simulink model "Refined_Model_3"  (R2020b)
settings: Solver=FixedStepAuto  StartTime=0.0  StopTime=90  FixedStep=dt  RelTol=1e-3
values from neighbouring files (symbols this model uses):
  CovDist = RoadProfile(:,4)    [ICE_Val.m]
  Cx = VehicleDefine(7,3)    [BEV_Basictest.m]    (also in GPS_val.m; ICEBEV_Script.m; ICEBEV_Script_VECTO.m; ICE_Script.m)
  DynRolRad = VehicleDefine(5,3)    [BEV_Basictest.m]    (also in GPS_val.m; ICEBEV_Script.m; ICEBEV_Script_VECTO.m; ICE_Script.m)
  EngineRpm = round(IntpTorCur(:,1))    [GPS_val.m]    (also in ICEBEV_Script.m; ICEBEV_Script_VECTO.m; ICE_Script.m; ICE_Script_SSVal.m)
  etaClutch = VehicleDefine(23,3)    [GPS_val.m]    (also in ICEBEV_Script.m; ICEBEV_Script_VECTO.m; ICE_Script.m; ICE_Script_SSVal.m)
  etaGRa = GBXDefine(:,3)    [GPS_val.m]    (also in ICEBEV_Script.m; ICEBEV_Script_VECTO.m; ICE_Script.m; ICE_Script_SSVal.m)
  FCTableVal = FCMap(2:end,2:end)    [GPS_val.m]    (also in ICEBEV_Script.m; ICEBEV_Script_VECTO.m; ICE_Script.m; ICE_Script_SSVal.m)
  FDR = VehicleDefine(20,3)    [BEV_Basictest.m]    (also in GPS_val.m = VehicleDefine(22,3); ICEBEV_Script.m = VehicleDefine(22,3); ICEBEV_Script_VECTO.m = VehicleDefine(22,3); ICE_Script.m = VehicleDefine(22,3))
  FLoadTor = IntpTorCur(:,2)    [GPS_val.m]    (also in ICEBEV_Script.m; ICEBEV_Script_VECTO.m; ICE_Script.m; ICE_Script_SSVal.m)
  Fr = VehicleDefine(13,3)    [BEV_Basictest.m]    (also in GPS_val.m; ICEBEV_Script.m; ICEBEV_Script_VECTO.m; ICE_Script.m)
  g = VehicleDefine(14,3)    [BEV_Basictest.m]    (also in GPS_val.m; ICEBEV_Script.m; ICEBEV_Script_VECTO.m; ICE_Script.m)
  GNo = GBXDefine(:,1)    [GPS_val.m]    (also in ICEBEV_Script.m; ICEBEV_Script_VECTO.m; ICE_Script.m; ICE_Script_SSVal.m)
  GRa = GBXDefine(:,2)    [GPS_val.m]    (also in ICEBEV_Script.m; ICEBEV_Script_VECTO.m; ICE_Script.m; ICE_Script_SSVal.m)
  InitVel = VehicleDefine(21,3)    [BEV_Basictest.m]    (also in GPS_val.m = VehicleDefine(24,3); ICEBEV_Script.m = VehicleDefine(24,3); ICEBEV_Script_VECTO.m = VehicleDefine(24,3); ICE_Script.m = VehicleDefine(24,3))
  IntpSlope = round(IntpSlope,1)    [GPS_val.m]    (also in ICE_Script.m; ICE_Val.m = A)
  Je = VehicleDefine(25,3)    [GPS_val.m]    (also in ICEBEV_Script.m; ICEBEV_Script_VECTO.m; ICE_Script.m; ICE_Script_SSVal.m)
  Jk = VehicleDefine(15,3)    [BEV_Basictest.m]    (also in GPS_val.m; ICEBEV_Script.m; ICEBEV_Script_VECTO.m; ICE_Script.m)
  Jm = VehicleDefine(16,3)    [GPS_val.m]    (also in ICEBEV_Script.m; ICEBEV_Script_VECTO.m; ICE_Script.m; ICE_Script_SSVal.m)
  MaxDec = 1    [BEV_Basictest.m]    (also in GPS_val.m; ICEBEV_Script.m; ICEBEV_Script_VECTO.m; ICE_Script.m)
  MaxSpeedProfile = FMSP    [GPS_val.m]    (also in ICE_Script.m; ICE_Val.m = repelem(SegSPLatinmps,SegLeninm))
  Me = VehicleDefine(10,3)    [BEV_Basictest.m]    (also in GPS_val.m; ICEBEV_Script.m; ICEBEV_Script_VECTO.m; ICE_Script.m)
  MotoringTor = IntpTorCur(:,3)    [GPS_val.m]    (also in ICEBEV_Script.m; ICEBEV_Script_VECTO.m; ICE_Script.m; ICE_Script_SSVal.m)
  Mt = VehicleDefine(12,3)    [BEV_Basictest.m]    (also in GPS_val.m; ICEBEV_Script.m; ICEBEV_Script_VECTO.m; ICE_Script.m)
  Mtot = Mv+Me+Mt    [BEV_Basictest.m]    (also in GPS_val.m; ICEBEV_Script.m; ICEBEV_Script_VECTO.m; ICE_Script.m)
  Mv = VehicleDefine(9,3)    [BEV_Basictest.m]    (also in GPS_val.m; ICEBEV_Script.m; ICEBEV_Script_VECTO.m; ICE_Script.m)
  NoSteps = round(Dist(end))    [GPS_val.m]    (also in ICE_Script.m; ICE_Val.m = 3002)
  NoWhlFA = VehicleDefine(2,3)    [BEV_Basictest.m]    (also in GPS_val.m; ICE_Script.m; ICE_Val.m; ICE_Val_new.m)
  NoWhlRA = VehicleDefine(4,3)    [BEV_Basictest.m]    (also in GPS_val.m; ICE_Script.m; ICE_Val.m; ICE_Val_new.m)
  rho = VehicleDefine(6,3)    [BEV_Basictest.m]    (also in GPS_val.m; ICEBEV_Script.m; ICEBEV_Script_VECTO.m; ICE_Script.m)
  RpmBrkPnt = ThrottleMap(1,:)    [GPS_val.m]    (also in ICEBEV_Script.m; ICEBEV_Script_VECTO.m; ICE_Script.m; ICE_Script_SSVal.m)
  s = divisors(length(MaxSpeedProfile))    [GPS_val.m]    (also in ICEBEV_Script.m = round(FLoadTor); ICEBEV_Script_VECTO.m = round(FLoadTor); ICE_Script.m = round(FLoadTor); ICE_Script_SSVal.m = round(FLoadTor))
  SegNo = RoadProfile(:,1)    [ICE_Val.m]
  SegSPLatinmps = (sqrt(aMaxLat*g*CurRadinm))    [GPS_val.m]    (also in ICE_Script.m; ICE_Val.m)
  Sx = VehicleDefine(8,3)    [BEV_Basictest.m]    (also in GPS_val.m; ICEBEV_Script.m; ICEBEV_Script_VECTO.m; ICE_Script.m)
  ThrotPos = ThrotPos'    [GPS_val.m]    (also in ICEBEV_Script.m; ICEBEV_Script_VECTO.m; ICE_Script.m; ICE_Script_SSVal.m)
  ThrotTableVal = ThrottleMap(2:end,2:end)    [GPS_val.m]    (also in ICEBEV_Script.m; ICEBEV_Script_VECTO.m; ICE_Script.m; ICE_Script_SSVal.m)
undefined symbols (not defined in the file or in its folder): Ftractive, G1Inprpm, GearNo, GInprpm, GInpTor, GTorLoss, MaxSpinG, MaxWhlTorinG
libraries: simulink x4, simulink_extras x2, autolibshared x1
settings Model: Creator=Kshitij  LastModifiedBy=Kshitij
settings DebuggingCC: AlgebraicLoopMsg=none

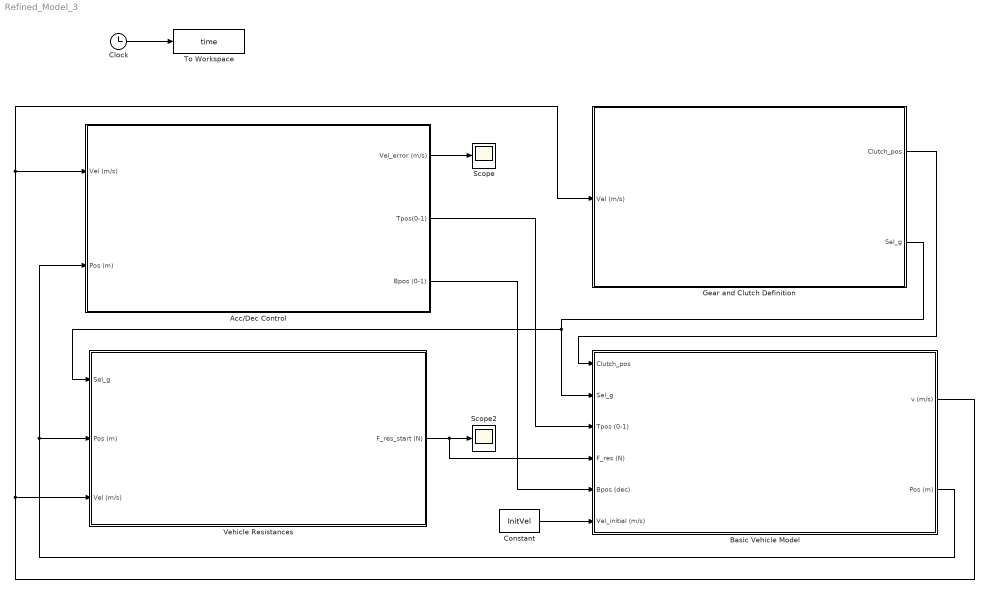
== system Refined_Model_3 ==
  Acc/Dec Control : Subsystem
  Basic Vehicle Model : Subsystem
  Clock : Clock
  Constant : Constant  Value=InitVel
  Gear and Clutch Definition : Subsystem
  Scope : Scope
  Scope2 : Scope
  To Workspace : ToWorkspace  VariableName=time  SaveFormat=Timeseries  SampleTime=-1
  Vehicle Resistances : Subsystem
  wires:
  Vehicle Resistances/1(F_res_start (N)) -> Basic Vehicle Model/4(F_res (N)), Scope2/1
  Basic Vehicle Model/2(Pos (m)) -> Acc/Dec Control/2(Pos (m)), Vehicle Resistances/2(Pos (m))
  Basic Vehicle Model/1(v (m/s)) -> Vehicle Resistances/3(Vel (m/s)), Gear and Clutch Definition/1(Vel (m/s)), Acc/Dec Control/1(Vel (m/s))
  Constant/1 -> Basic Vehicle Model/6(Vel_initial (m/s))
  Acc/Dec Control/1(Vel_error (m/s)) -> Scope/1
  Gear and Clutch Definition/2(Sel_g) -> Basic Vehicle Model/2(Sel_g), Vehicle Resistances/1(Sel_g)
  Gear and Clutch Definition/1(Clutch_pos) -> Basic Vehicle Model/1(Clutch_pos)
  Clock/1 -> To Workspace/1
  Acc/Dec Control/2(Tpos(0-1)) -> Basic Vehicle Model/3(Tpos (0-1))
  Acc/Dec Control/3(Bpos (0-1)) -> Basic Vehicle Model/5(Bpos (dec))

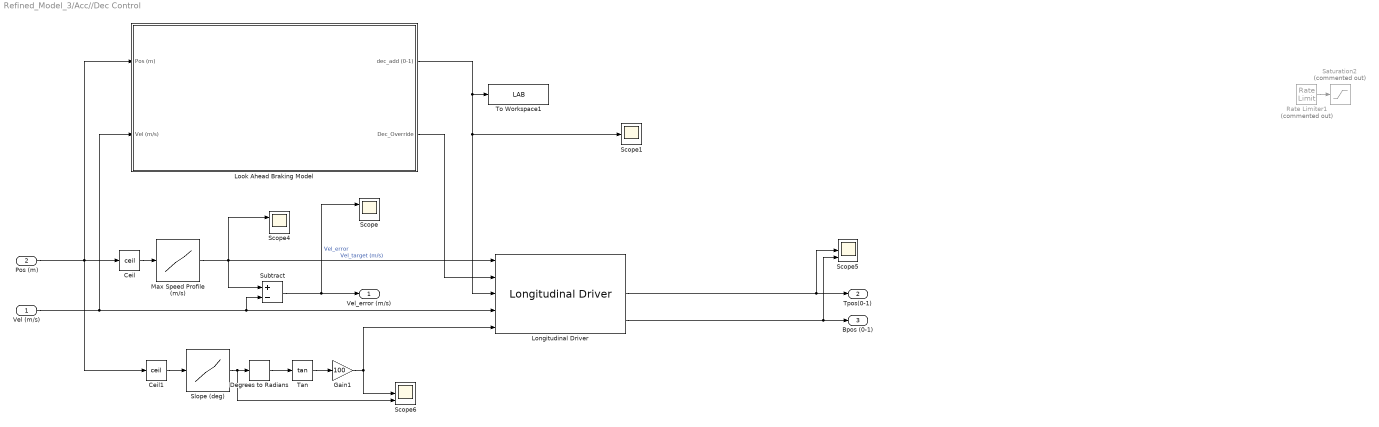
== system Refined_Model_3/Acc//Dec Control ==
  Vel (m/s) : Inport
  Pos (m) : Inport  Port=2
  Ceil : Rounding  Operator=ceil
  Ceil1 : Rounding  Operator=ceil
  Degrees to Radians : simulink_extras/Transformations/Degrees to Radians
  Gain1 : Gain  Gain=100
  Longitudinal Driver : autolibshared/Longitudinal Driver  extAccelOvr=off  extDecelOvr=on  extAccelHld=off  extDecelHld=off  extAccelZero=off  extDecelZero=off  cntrlType=PI  shftType=None  velUnits=m/s  gearOut=off  Kp=10  Ki=20  Kff=.05  Kg=.01  VehVelVec=[0 100]  KffVec=[.1 .1]  KpVec=[10 10]  KiVec=[5 5]  KgVec=[0 0]  m=1500  Kpt=3000  tau=.1  L=2  aR=200  bR=2.5  cR=.5  g=9.81  vnom=100  Kaw=.1  tauerr=.03  tauPt=2  GearInit=0  tShift=.1  pdlVec=[0.1 0.4 0.5 0.9]  upShftTbl=[-1 12.9375 26.4375 39.9375 51.18749999999999 62.4375 72.84375 83.25;-1 16.3125 29.8125 43.3125 54.5624 65.8125 76.78125 87.75;-1 19.6875 33.1875 46.68749999999999 57.9375 69.1875 80.71875 92.25;-1 33 52.5 77.25 100.5 138.75 161.875 185]  dwnShftTbl=[1 9.5625 23.0625 36.5625 47.8125 59.0625 68.90625 78.75;1 12.9375 26.4375 39.9375 51.18749999999999 62.4375 72.84375 83.25;1 16.3125 29.8125 43.3125 54.562499 65.8125 76.78125 87.75;1 19.6875 33.1875 46.68749999999999 57.9375 69.1875 80.71875 92.25]  tClutch=.5  tRev=.5  tPark=120  aMode=1  UpGearVec="[0  1  2  3  4  5  6  7]"  DownGearVec="[1  2  3  4  5  6  7  8]"
      settings: SourceProductBaseCode=PW,MT,UV,VE,VP
  Look Ahead Braking Model : Subsystem
  Max Speed Profile (m/s) : Lookup_n-D  NumberOfTableDimensions=1  BreakpointsForDimension1=[1:length(MaxSpeedProfile)]  BreakpointsForDimension2=G1Inprpm  Table=MaxSpeedProfile  InterpMethod=Linear Lagrange  InternalRulePriority=Speed  RndMeth=Simplest  InputSameDT=on
  Rate Limiter1 : RateLimiter  Commented=on  RisingSlewLimit=0.5  FallingSlewLimit=-0.5  SampleTimeMode=inherited
  Saturation2 : Saturate  Commented=on  UpperLimit=1  LowerLimit=-1
  Scope : Scope  NumInputPorts=2
  Scope1 : Scope
  Scope4 : Scope  NumInputPorts=2
  Scope5 : Scope  NumInputPorts=3
  Scope6 : Scope  NumInputPorts=3
  Slope (deg) : Lookup_n-D  NumberOfTableDimensions=1  BreakpointsForDimension1=1: length(IntpSlope)  Table=IntpSlope  InternalRulePriority=Speed  RndMeth=Simplest  InputSameDT=on
  Subtract : Sum  Inputs=+-
  Tan : Trigonometry  Operator=tan
  To Workspace1 : ToWorkspace  VariableName=LAB  SaveFormat=Timeseries  SampleTime=-1
  Vel_error (m/s) : Outport
  Tpos(0-1) : Outport  Port=2
  Bpos (0-1) : Outport  Port=3
  wires:
  Max Speed Profile (m/s)/1 -> Subtract/1, Longitudinal Driver/1, Scope4/1  "Vel_target (m/s)"
  Subtract/1 -> Scope/1, Vel_error (m/s)/1  "Vel_error"
  Ceil/1 -> Max Speed Profile (m/s)/1
  Look Ahead Braking Model/1(dec_add (0-1)) -> Longitudinal Driver/3, Scope1/1, To Workspace1/1
  Pos (m)/1 -> Ceil1/1, Ceil/1, Look Ahead Braking Model/1(Pos (m))
  Rate Limiter1/1 -> Saturation2/1
  Vel (m/s)/1 -> Longitudinal Driver/4, Subtract/2, Look Ahead Braking Model/2(Vel (m/s))
  Slope (deg)/1 -> Scope6/3, Degrees to Radians/1
  Ceil1/1 -> Slope (deg)/1
  Degrees to Radians/1 -> Tan/1
  Tan/1 -> Gain1/1
  Gain1/1 -> Scope6/2, Longitudinal Driver/5
  Longitudinal Driver/2 -> Scope5/2, Tpos(0-1)/1
  Longitudinal Driver/3 -> Scope5/3, Bpos (0-1)/1
  Look Ahead Braking Model/2(Dec_Override) -> Longitudinal Driver/2

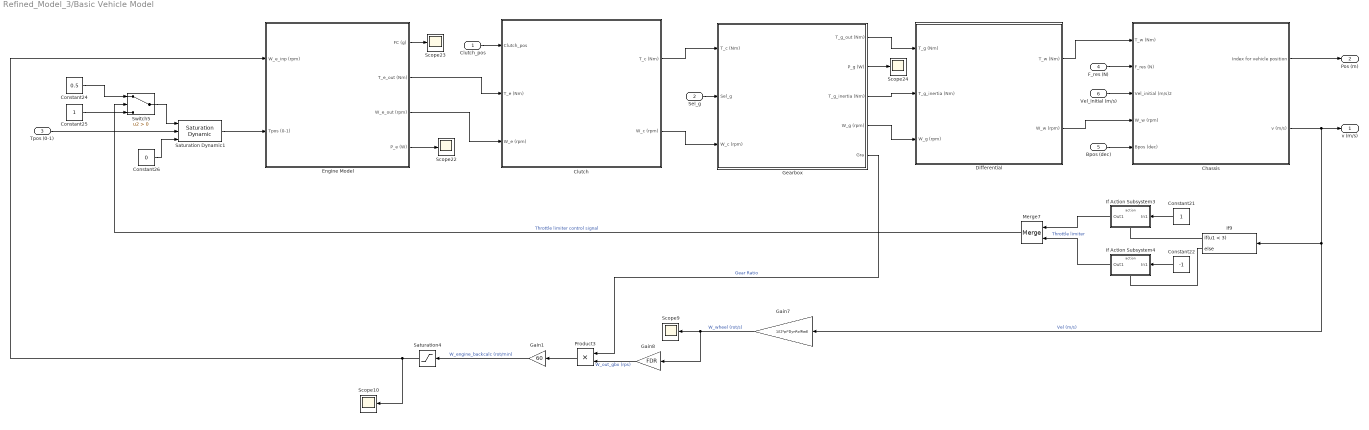
== system Refined_Model_3/Basic Vehicle Model ==
  Clutch_pos : Inport
  Sel_g : Inport  Port=2
  Tpos (0-1) : Inport  Port=3
  F_res (N) : Inport  Port=4
  Bpos (dec) : Inport  Port=5
  Vel_initial (m/s) : Inport  Port=6
  Chassis : Subsystem
  Clutch : Subsystem
  Constant21 : Constant
  Constant22 : Constant  Value=-1
  Constant24 : Constant  Value=0.5
  Constant25 : Constant
  Constant26 : Constant  Value=0
  Differential : Subsystem
  Engine Model : Subsystem
  Gain1 : Gain  Gain=60
  Gain7 : Gain  Gain=1/(2*pi*DynRolRad)
  Gain8 : Gain  Gain=FDR
  Gearbox : Subsystem
  If Action Subsystem3 : Subsystem  TreatAsAtomicUnit=on
  If Action Subsystem4 : Subsystem  TreatAsAtomicUnit=on
  If9 : If  IfExpression=u1 < 3
  Merge7 : Merge
  Product3 : Product
  Saturation Dynamic1 : simulink/Discontinuities/Saturation Dynamic  OutMin=[]  OutMax=[]  OutDataTypeStr=Inherit: Same as second input  OutDataType=fixdt(1, 16)  OutScaling=2^-10  DoSatur=off
  Saturation4 : Saturate  UpperLimit=max(EngineRpm)  LowerLimit=min(EngineRpm)
  Scope{9..10,22..24} (5 alike) : Scope
  Switch5 : Switch  Criteria=u2 > Threshold
  v (m/s) : Outport
  Pos (m) : Outport  Port=2
  wires:
  Gearbox/1(T_g_out (Nm)) -> Differential/1(T_g (Nm))
  Gearbox/4(W_g (rpm)) -> Differential/3(W_g (rpm))
  Gearbox/3(T_g_inertia (Nm)) -> Differential/2(T_g_inertia (Nm))
  Chassis/1(Index for vehicle position) -> Pos (m)/1
  Bpos (dec)/1 -> Chassis/5(Bpos (dec))
  Vel_initial (m/s)/1 -> Chassis/3(Vel_initial (m/s)2)
  Differential/1(T_w (Nm)) -> Chassis/1(T_w (Nm))
  F_res (N)/1 -> Chassis/2(F_res (N))
  Constant21/1 -> If Action Subsystem3/1(In1)
  If9/1 -> If Action Subsystem3/Action
  Gearbox/2(P_g (W)) -> Scope24/1
  Clutch/1(T_c (Nm)) -> Gearbox/1(T_c (Nm))
  Clutch/2(W_c (rpm)) -> Gearbox/3(W_c (rpm))
  Saturation Dynamic1/1 -> Engine Model/2(Tpos (0-1))
  Tpos (0-1)/1 -> Saturation Dynamic1/2
  Merge7/1 -> Switch5/2  "Throttle limiter control signal"
  Constant26/1 -> Saturation Dynamic1/3
  Constant24/1 -> Switch5/1
  Engine Model/4(P_e (W)) -> Scope22/1
  Constant25/1 -> Switch5/3
  If Action Subsystem3/1(Out1) -> Merge7/1
  Switch5/1 -> Saturation Dynamic1/1
  Differential/2(W_w (rpm)) -> Chassis/4(W_w (rpm))
  Engine Model/2(T_e_out (Nm)) -> Clutch/2(T_e (Nm))
  Engine Model/1(FC (g)) -> Scope23/1
  Sel_g/1 -> Gearbox/2(Sel_g)
  If9/2 -> If Action Subsystem4/Action
  Engine Model/3(W_e_out (rpm)) -> Clutch/3(W_e (rpm))
  If Action Subsystem4/1(Out1) -> Merge7/2  "Throttle limiter"
  Clutch_pos/1 -> Clutch/1(Clutch_pos)
  Constant22/1 -> If Action Subsystem4/1(In1)
  Gain1/1 -> Saturation4/1  "W_engine_backcalc (rot/min)"
  Gain7/1 -> Scope9/1, Gain8/1  "W_wheel (rot/s)"
  Chassis/2(v (m/s)) -> v (m/s)/1, Gain7/1, If9/1  "Vel (m/s)"
  Gearbox/5(Gra) -> Product3/1  "Gear Ratio"
  Product3/1 -> Gain1/1
  Gain8/1 -> Product3/2  "W_out_gbx (rps)"
  Saturation4/1 -> Scope10/1, Engine Model/1(W_e_inp (rpm))

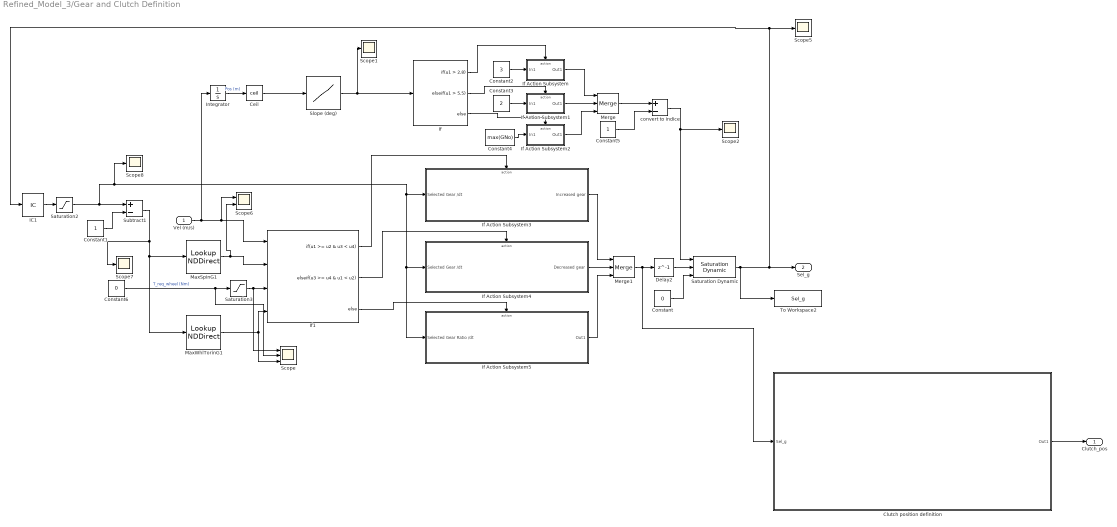
== system Refined_Model_3/Gear and Clutch Definition ==
  Vel (m/s) : Inport
  Ceil : Rounding  Operator=ceil
  Clutch position definition : Subsystem
  Constant : Constant  Value=0
  Constant1 : Constant
  Constant2 : Constant  Value=3
  Constant3 : Constant  Value=2
  Constant4 : Constant  Value=max(GNo)
  Constant5 : Constant
  Constant6 : Constant  Value=0
  Delay2 : Delay  DelayLength=1
  IC1 : InitialCondition
  If : If  IfExpression=u1 > 2.8  ElseIfExpressions=u1 > 5.5
  If Action Subsystem : Subsystem  TreatAsAtomicUnit=on
  If Action Subsystem1 : Subsystem  TreatAsAtomicUnit=on
  If Action Subsystem2 : Subsystem  TreatAsAtomicUnit=on
  If Action Subsystem3 : Subsystem  TreatAsAtomicUnit=on
  If Action Subsystem4 : Subsystem  TreatAsAtomicUnit=on
  If Action Subsystem5 : Subsystem  TreatAsAtomicUnit=on
  If1 : If  NumInputs=4  IfExpression=u1 >= u2 & u3 < u4  ElseIfExpressions=u3 >= u4 & u1 < u2
  Integrator : Integrator
  MaxSpinG1 : LookupNDDirect  NumberOfTableDimensions=1  Table=MaxSpinG
  MaxWhlTorinG1 : LookupNDDirect  NumberOfTableDimensions=1  Table=MaxWhlTorinG
  Merge : Merge  Inputs=3
  Merge1 : Merge  Inputs=3
  Saturation Dynamic : simulink/Discontinuities/Saturation Dynamic  OutMin=[]  OutMax=[]  OutDataTypeStr=Inherit: Same as second input  OutDataType=fixdt(1, 16)  OutScaling=2^-10  DoSatur=off
  Saturation2 : Saturate  UpperLimit=max(GNo)  LowerLimit=0
  Saturation3 : Saturate  UpperLimit=inf  LowerLimit=0
  Scope : Scope  NumInputPorts=3
  Scope{1..2,5,7..8} (5 alike) : Scope
  Scope6 : Scope  NumInputPorts=2
  Slope (deg) : Lookup_n-D  NumberOfTableDimensions=1  BreakpointsForDimension1=1: length(IntpSlope)  Table=IntpSlope  InternalRulePriority=Speed  RndMeth=Simplest  InputSameDT=on
  Subtract1 : Sum  Inputs=+-
  To Workspace2 : ToWorkspace  VariableName=Sel_g  SaveFormat=Timeseries  SampleTime=-1
  convert to indice : Sum  Inputs=+-
  Clutch_pos : Outport
  Sel_g : Outport  Port=2
  wires:
  IC1/1 -> Saturation2/1
  Merge1/1 -> Clutch position definition/1(Sel_g), Delay2/1
  Clutch position definition/1(Out1) -> Clutch_pos/1
  If1/2 -> If Action Subsystem4/Action
  If Action Subsystem4/1(Decreased gear) -> Merge1/2
  If1/3 -> If Action Subsystem5/Action
  If Action Subsystem3/1(Increased gear) -> Merge1/1
  Constant1/1 -> Subtract1/2
  MaxSpinG1/1 -> Scope6/2, If1/2
  If Action Subsystem5/1(Out1) -> Merge1/3
  Subtract1/1 -> Scope7/1, MaxSpinG1/1, MaxWhlTorinG1/1
  MaxWhlTorinG1/1 -> Scope/3, If1/4
  Saturation2/1 -> Subtract1/1, If Action Subsystem5/1(Selected Gear Ratio /dt), If Action Subsystem4/1(Selected Gear /dt), If Action Subsystem3/1(Selected Gear /dt), Scope8/1
  Vel (m/s)/1 -> If1/1, Scope6/1, Integrator/1
  If1/1 -> If Action Subsystem3/Action
  Saturation3/1 -> If1/3, Scope/1
  Integrator/1 -> Ceil/1  "Pos (m)"
  Ceil/1 -> Slope (deg)/1
  Slope (deg)/1 -> Scope1/1, If/1
  If/1 -> If Action Subsystem/Action
  If/2 -> If Action Subsystem1/Action
  Constant/1 -> Saturation Dynamic/3
  Constant2/1 -> If Action Subsystem/1(In1)
  If Action Subsystem/1(Out1) -> Merge/1
  If Action Subsystem1/1(Out1) -> Merge/2
  If/3 -> If Action Subsystem2/Action
  Constant3/1 -> If Action Subsystem1/1(In1)
  Constant4/1 -> If Action Subsystem2/1(In1)
  If Action Subsystem2/1(Out1) -> Merge/3
  convert to indice/1 -> Scope2/1, Saturation Dynamic/1
  Saturation Dynamic/1 -> To Workspace2/1, Sel_g/1, IC1/1, Scope5/1
  Delay2/1 -> Saturation Dynamic/2
  Merge/1 -> convert to indice/1
  Constant5/1 -> convert to indice/2
  Constant6/1 -> Scope/2, Saturation3/1  "T_req_wheel (Nm)"

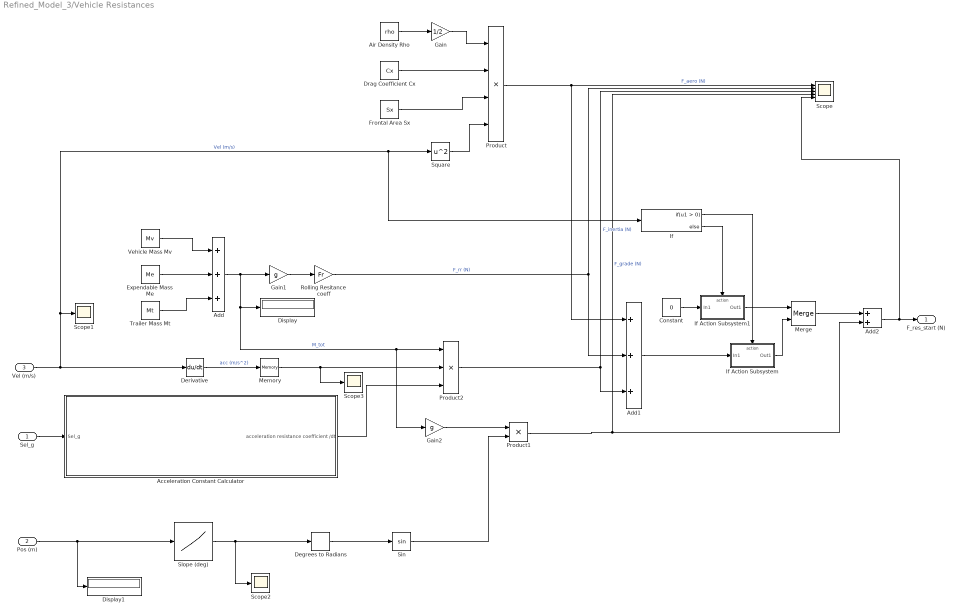
== system Refined_Model_3/Vehicle Resistances ==
  Sel_g : Inport
  Pos (m) : Inport  Port=2
  Vel (m/s) : Inport  Port=3
  Acceleration Constant Calculator : Subsystem
  Add : Sum  Inputs=+++
  Add1 : Sum  Inputs=+++
  Add2 : Sum
  Air Density Rho : Constant  Value=rho
  Constant : Constant  Value=0
  Degrees to Radians : simulink_extras/Transformations/Degrees to Radians
  Derivative : Derivative
  Display : Display
  Display1 : Display
  Drag Coefficient Cx : Constant  Value=Cx
  Expendable Mass Me : Constant  Value=Me
  Frontal Area Sx : Constant  Value=Sx
  Gain : Gain  Gain=1/2
  Gain1 : Gain  Gain=g
  Gain2 : Gain  Gain=g
  If : If
  If Action Subsystem : Subsystem  TreatAsAtomicUnit=on
  If Action Subsystem1 : Subsystem  TreatAsAtomicUnit=on
  Memory : Memory
  Merge : Merge
  Product : Product  Inputs=4
  Product1 : Product
  Product2 : Product  Inputs=3
  Rolling Resitance coeff : Gain  Gain=Fr
  Scope : Scope  NumInputPorts=5
  Scope1 : Scope
  Scope2 : Scope
  Scope3 : Scope
  Sin : Trigonometry
  Slope (deg) : Lookup_n-D  NumberOfTableDimensions=1  BreakpointsForDimension1=1: length(IntpSlope)  Table=IntpSlope  InternalRulePriority=Speed  RndMeth=Simplest  InputSameDT=on
  Square : Math  Operator=square  SaturateOnIntegerOverflow=on
  Trailer Mass Mt : Constant  Value=Mt
  Vehicle Mass Mv : Constant  Value=Mv
  F_res_start (N) : Outport
  wires:
  Expendable Mass Me/1 -> Add/2
  Add/1 -> Display/1, Product2/1, Gain2/1, Gain1/1  "M_tot"
  Gain/1 -> Product/1
  Sin/1 -> Product1/2
  Slope (deg)/1 -> Degrees to Radians/1, Scope2/1
  Product1/1 -> Add2/2, Scope/4  "F_grade (N)"
  Air Density Rho/1 -> Gain/1
  Drag Coefficient Cx/1 -> Product/2
  Vel (m/s)/1 -> Derivative/1, If/1, Square/1, Scope1/1  "Vel (m/s)"
  Pos (m)/1 -> Display1/1, Slope (deg)/1
  Gain2/1 -> Product1/1
  Trailer Mass Mt/1 -> Add/3
  Rolling Resitance coeff/1 -> Scope/2, Add1/2  "F_rr (N)"
  Square/1 -> Product/4
  Gain1/1 -> Rolling Resitance coeff/1
  Vehicle Mass Mv/1 -> Add/1
  Product/1 -> Add1/1, Scope/1  "F_aero (N)"
  Frontal Area Sx/1 -> Product/3
  Product2/1 -> Add1/3, Scope/3  "F_inertia (N)"
  Acceleration Constant Calculator/1(acceleration resistance coefficient /dt) -> Product2/3
  Sel_g/1 -> Acceleration Constant Calculator/1(Sel_g)
  Derivative/1 -> Memory/1  "acc (m/s^2)"
  If/1 -> If Action Subsystem/Action
  If/2 -> If Action Subsystem1/Action
  If Action Subsystem1/1(Out1) -> Merge/1
  Add1/1 -> If Action Subsystem/1(In1)
  If Action Subsystem/1(Out1) -> Merge/2
  Constant/1 -> If Action Subsystem1/1(In1)
  Merge/1 -> Add2/1
  Add2/1 -> Scope/5, F_res_start (N)/1
  Degrees to Radians/1 -> Sin/1
  Memory/1 -> Scope3/1, Product2/2

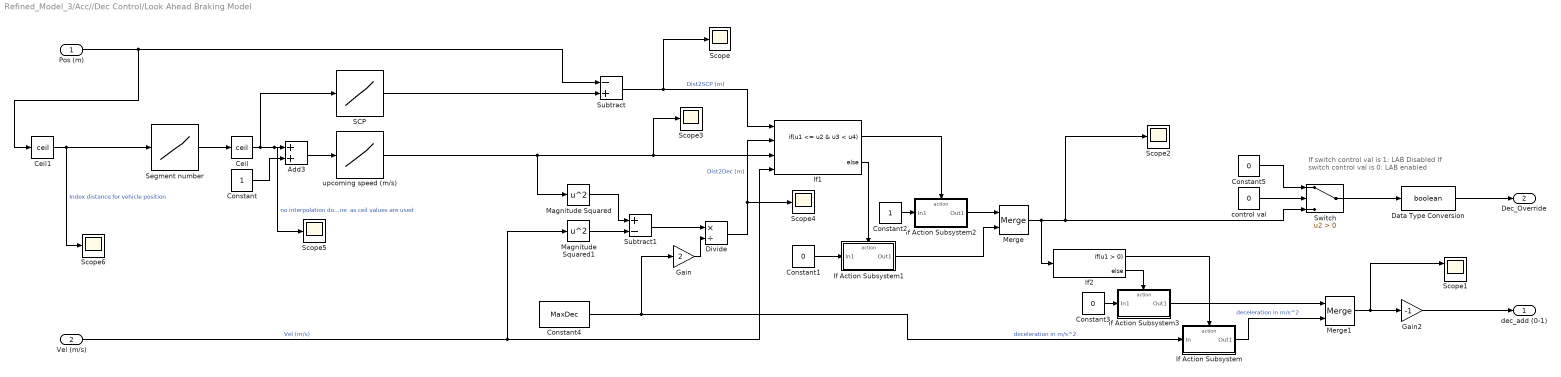
== system Refined_Model_3/Acc//Dec Control/Look Ahead Braking Model ==
  note: If switch control val is 1: LAB Disabled
      | If switch control val is 0: LAB enabled
  Pos (m) : Inport
  Vel (m/s) : Inport  Port=2
  Add3 : Sum
  Ceil : Rounding  Operator=ceil
  Ceil1 : Rounding  Operator=ceil
  Constant : Constant
  Constant1 : Constant  Value=0
  Constant2 : Constant
  Constant3 : Constant  Value=0
  Constant4 : Constant  Value=MaxDec
  Constant5 : Constant  Value=0
  Data Type Conversion : DataTypeConversion  OutDataTypeStr=boolean
  Divide : Product  Inputs=*/
  Gain : Gain  Gain=2
  Gain2 : Gain  Gain=-1
  If Action Subsystem : Subsystem  TreatAsAtomicUnit=on
  If Action Subsystem1 : Subsystem  TreatAsAtomicUnit=on
  If Action Subsystem2 : Subsystem  TreatAsAtomicUnit=on
  If Action Subsystem3 : Subsystem  TreatAsAtomicUnit=on
  If1 : If  NumInputs=4  IfExpression=u1 <= u2 & u3 < u4
  If2 : If
  Magnitude Squared : Math  Operator=square  SaturateOnIntegerOverflow=on
  Magnitude Squared1 : Math  Operator=square  SaturateOnIntegerOverflow=on
  Merge : Merge
  Merge1 : Merge
  SCP : Lookup_n-D  NumberOfTableDimensions=1  BreakpointsForDimension1=SegNo  BreakpointsForDimension2=G1Inprpm  Table=CovDist  InterpMethod=Linear Lagrange  InternalRulePriority=Speed  RndMeth=Simplest  InputSameDT=on
  Scope{,2..6} (6 alike) : Scope
  Scope1 : Scope  NumInputPorts=2
  Segment number : Lookup_n-D  NumberOfTableDimensions=1  BreakpointsForDimension1=CovDist  BreakpointsForDimension2=G1Inprpm  Table=SegNo  InterpMethod=Linear Lagrange  InternalRulePriority=Speed  RndMeth=Simplest  InputSameDT=on
  Subtract : Sum  Inputs=-+
  Subtract1 : Sum  Inputs=+-
  Switch : Switch  Criteria=u2 > Threshold
  control val : Constant  Value=0
  upcoming speed (m/s) : Lookup_n-D  NumberOfTableDimensions=1  BreakpointsForDimension1=SegNo  BreakpointsForDimension2=G1Inprpm  Table=SegSPLatinmps  InterpMethod=Linear Lagrange  InternalRulePriority=Speed  RndMeth=Simplest  InputSameDT=on
  dec_add (0-1) : Outport
  Dec_Override : Outport  Port=2
  wires:
  Add3/1 -> upcoming speed (m/s)/1
  Ceil/1 -> SCP/1, Scope5/1, Add3/1  "no interpolation done  as ceil values are used"
  SCP/1 -> Subtract/2
  upcoming speed (m/s)/1 -> Scope3/1, If1/3, Magnitude Squared/1
  Constant/1 -> Add3/2
  Subtract/1 -> Scope/1, If1/1  "Dist2SCP (m)"
  Segment number/1 -> Ceil/1
  Ceil1/1 -> Scope6/1, Segment number/1  "Index distance for vehicle position"
  Magnitude Squared/1 -> Subtract1/1
  Subtract1/1 -> Divide/1
  Gain/1 -> Divide/2
  Constant4/1 -> Gain/1, If Action Subsystem/1(In)  "deceleration in m/s^2"
  Divide/1 -> Scope4/1, If1/2  "Dist2Dec (m)"
  Vel (m/s)/1 -> Magnitude Squared1/1, If1/4  "Vel (m/s)"
  If Action Subsystem/1(Out1) -> Merge1/2  "deceleration in m/s^2"
  If1/2 -> If Action Subsystem1/Action
  Constant1/1 -> If Action Subsystem1/1(In1)
  Constant2/1 -> If Action Subsystem2/1(In1)
  If1/1 -> If Action Subsystem2/Action
  If Action Subsystem2/1(Out1) -> Merge/1
  If Action Subsystem1/1(Out1) -> Merge/2
  If2/1 -> If Action Subsystem/Action
  If2/2 -> If Action Subsystem3/Action
  Constant3/1 -> If Action Subsystem3/1(In1)
  If Action Subsystem3/1(Out1) -> Merge1/1
  Magnitude Squared1/1 -> Subtract1/2
  Pos (m)/1 -> Ceil1/1, Subtract/1
  Merge1/1 -> Gain2/1, Scope1/1
  control val/1 -> Switch/2
  Constant5/1 -> Switch/1
  Switch/1 -> Data Type Conversion/1
  Merge/1 -> If2/1, Switch/3, Scope2/1
  Data Type Conversion/1 -> Dec_Override/1
  Gain2/1 -> dec_add (0-1)/1

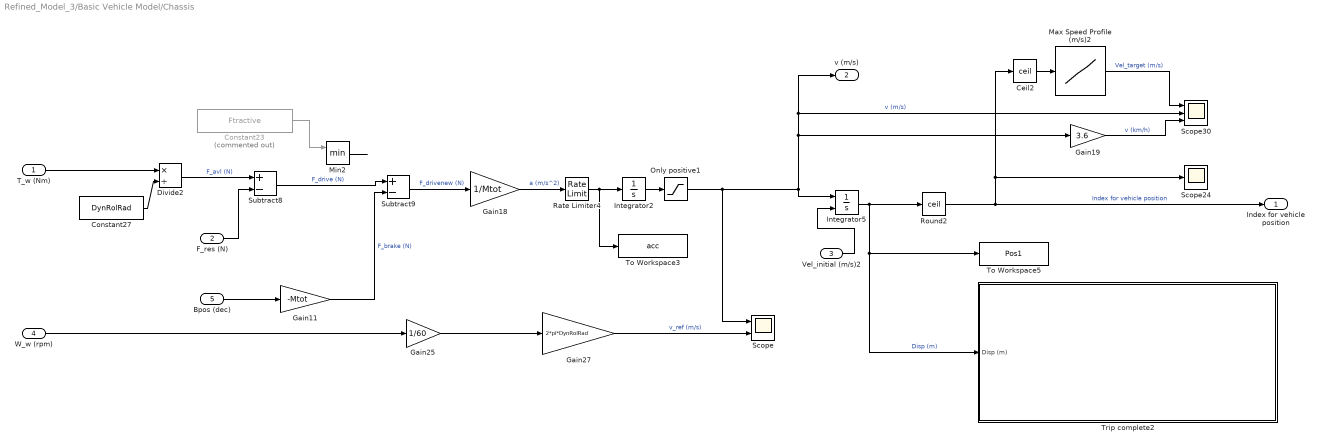
== system Refined_Model_3/Basic Vehicle Model/Chassis ==
  T_w (Nm) : Inport
  F_res (N) : Inport  Port=2
  Vel_initial (m/s)2 : Inport  Port=3
  W_w (rpm) : Inport  Port=4
  Bpos (dec) : Inport  Port=5
  Ceil2 : Rounding  Operator=ceil
  Constant23 : Constant  Commented=on  Value=Ftractive
  Constant27 : Constant  Value=DynRolRad
  Divide2 : Product  Inputs=*/
  Gain11 : Gain  Gain=-Mtot
  Gain18 : Gain  Gain=1/Mtot
  Gain19 : Gain  Gain=3.6
  Gain25 : Gain  Gain=1/60
  Gain27 : Gain  Gain=2*pi*DynRolRad
  Integrator2 : Integrator  ContinuousStateAttributes='acceleration'
  Integrator5 : Integrator  InitialConditionSource=external  ContinuousStateAttributes='velocity'
  Max Speed Profile (m/s)2 : Lookup_n-D  NumberOfTableDimensions=1  BreakpointsForDimension1=[1:length(MaxSpeedProfile)]  BreakpointsForDimension2=G1Inprpm  Table=MaxSpeedProfile  InterpMethod=Linear Lagrange  InternalRulePriority=Speed  RndMeth=Simplest  InputSameDT=on
  Min2 : MinMax  Inputs=2
  Only positive1 : Saturate  UpperLimit=inf  LowerLimit=0
  Rate Limiter4 : RateLimiter  RisingSlewLimit=0.5  FallingSlewLimit=-0.5  SampleTimeMode=inherited
  Round2 : Rounding  Operator=ceil
  Scope : Scope  NumInputPorts=2
  Scope24 : Scope
  Scope30 : Scope  NumInputPorts=3
  Subtract8 : Sum  Inputs=+-
  Subtract9 : Sum  Inputs=+-
  To Workspace3 : ToWorkspace  VariableName=acc  SaveFormat=Timeseries  SampleTime=-1
  To Workspace5 : ToWorkspace  VariableName=Pos1  SaveFormat=Timeseries  SampleTime=-1
  Trip complete2 : Subsystem
  Index for vehicle position : Outport
  v (m/s) : Outport  Port=2
  wires:
  W_w (rpm)/1 -> Gain25/1
  Rate Limiter4/1 -> Integrator2/1, To Workspace3/1
  Constant27/1 -> Divide2/2
  Subtract9/1 -> Gain18/1  "F_drivenew (N)"
  Subtract8/1 -> Subtract9/1  "F_drive (N)"
  Divide2/1 -> Subtract8/1  "F_avl (N)"
  Integrator5/1 -> Round2/1, To Workspace5/1, Trip complete2/1(Disp (m))  "Disp (m)"
  Min2/1 -> ?
  Ceil2/1 -> Max Speed Profile (m/s)2/1
  Integrator2/1 -> Only positive1/1
  T_w (Nm)/1 -> Divide2/1
  Gain11/1 -> Subtract9/2  "F_brake (N)"
  Round2/1 -> Index for vehicle position/1, Ceil2/1, Scope24/1  "Index for vehicle position"
  F_res (N)/1 -> Subtract8/2
  Only positive1/1 -> Scope/1, Integrator5/1, v (m/s)/1, Scope30/2, Gain19/1  "v (m/s)"
  Vel_initial (m/s)2/1 -> Integrator5/2
  Gain27/1 -> Scope/2  "v_ref (m/s)"
  Gain19/1 -> Scope30/3  "v (km/h)"
  Constant23/1 -> Min2/1
  Max Speed Profile (m/s)2/1 -> Scope30/1  "Vel_target (m/s)"
  Gain18/1 -> Rate Limiter4/1  "a (m/s^2)"
  Gain25/1 -> Gain27/1
  Bpos (dec)/1 -> Gain11/1

== system Refined_Model_3/Basic Vehicle Model/Clutch ==
  Clutch_pos : Inport
  T_e (Nm) : Inport  Port=2
  W_e (rpm) : Inport  Port=3
  Clutch value1 : Product
  Gain20 : Gain  Gain=etaClutch
  IC2 : InitialCondition  Value=0
  Product9 : Product
  Saturation3 : Saturate  UpperLimit=1  LowerLimit=0.5
  Scope : Scope
  Scope1 : Scope
  Scope27 : Scope
  T_c (Nm) : Outport
  W_c (rpm) : Outport  Port=2
  wires:
  IC2/1 -> Saturation3/1, Clutch value1/1
  Saturation3/1 -> Product9/1
  Clutch value1/1 -> Gain20/1, Scope27/1
  Clutch_pos/1 -> IC2/1
  T_e (Nm)/1 -> Clutch value1/2
  Product9/1 -> Scope1/1, W_c (rpm)/1  "W_c (rpm)"
  Gain20/1 -> Scope/1, T_c (Nm)/1  "T_c (Nm)"
  W_e (rpm)/1 -> Product9/2

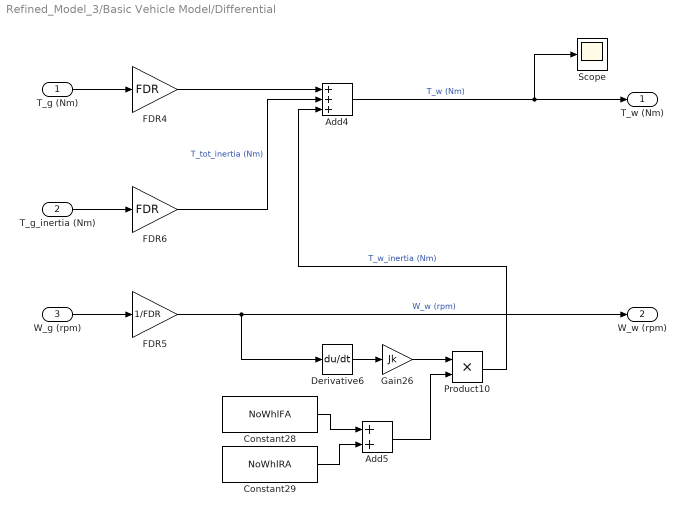
== system Refined_Model_3/Basic Vehicle Model/Differential ==
  T_g (Nm) : Inport
  T_g_inertia (Nm) : Inport  Port=2
  W_g (rpm) : Inport  Port=3
  Add4 : Sum  Inputs=+++
  Add5 : Sum
  Constant28 : Constant  Value=NoWhlFA
  Constant29 : Constant  Value=NoWhlRA
  Derivative6 : Derivative
  FDR4 : Gain  Gain=FDR
  FDR5 : Gain  Gain=1/FDR
  FDR6 : Gain  Gain=FDR
  Gain26 : Gain  Gain=Jk
  Product10 : Product
  Scope : Scope
  T_w (Nm) : Outport
  W_w (rpm) : Outport  Port=2
  wires:
  Product10/1 -> Add4/3  "T_w_inertia (Nm)"
  Derivative6/1 -> Gain26/1
  Add5/1 -> Product10/2
  Constant29/1 -> Add5/2
  FDR6/1 -> Add4/2  "T_tot_inertia (Nm)"
  Constant28/1 -> Add5/1
  FDR4/1 -> Add4/1
  FDR5/1 -> Derivative6/1, W_w (rpm)/1  "W_w (rpm)"
  Gain26/1 -> Product10/1
  T_g_inertia (Nm)/1 -> FDR6/1
  Add4/1 -> Scope/1, T_w (Nm)/1  "T_w (Nm)"
  T_g (Nm)/1 -> FDR4/1
  W_g (rpm)/1 -> FDR5/1

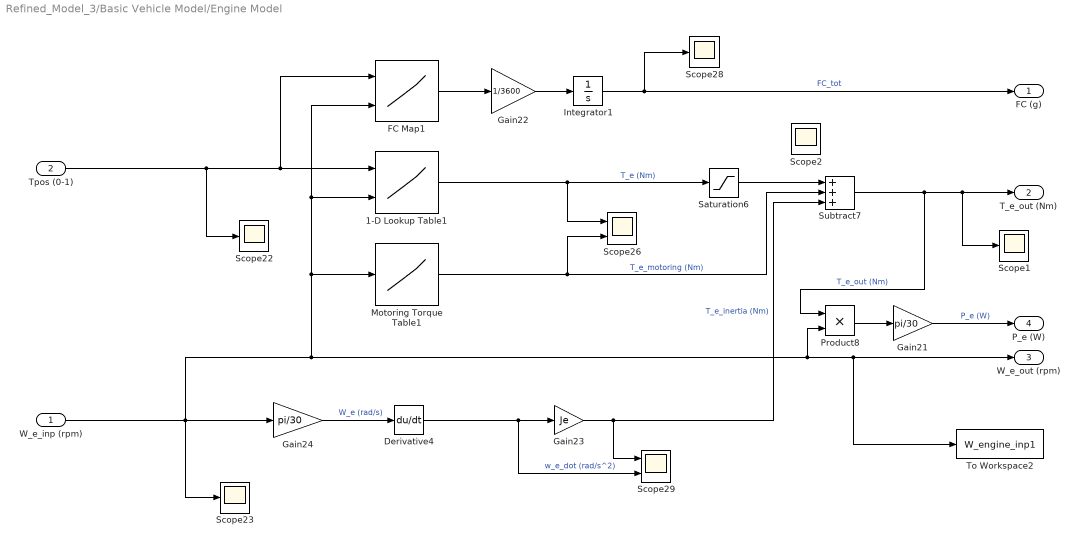
== system Refined_Model_3/Basic Vehicle Model/Engine Model ==
  W_e_inp (rpm) : Inport
  Tpos (0-1) : Inport  Port=2
  1-D Lookup Table1 : Lookup_n-D  BreakpointsForDimension1=ThrotPos  BreakpointsForDimension2=RpmBrkPnt  Table=ThrotTableVal  InternalRulePriority=Speed  RndMeth=Simplest  InputSameDT=on
      settings: InputPortMap=u0,u1
  Derivative4 : Derivative
  FC Map1 : Lookup_n-D  BreakpointsForDimension1=ThrotPos  BreakpointsForDimension2=RpmBrkPnt  Table=FCTableVal  InternalRulePriority=Speed  RndMeth=Simplest  InputSameDT=on
      settings: InputPortMap=u0,u1
  Gain21 : Gain  Gain=pi/30
  Gain22 : Gain  Gain=1/3600
  Gain23 : Gain  Gain=Je
  Gain24 : Gain  Gain=pi/30
  Integrator1 : Integrator
  Motoring Torque Table1 : Lookup_n-D  NumberOfTableDimensions=1  BreakpointsForDimension1=EngineRpm  BreakpointsForDimension2=G1Inprpm  Table=MotoringTor  InterpMethod=Linear Lagrange  InternalRulePriority=Speed  RndMeth=Simplest  InputSameDT=on
  Product8 : Product
  Saturation6 : Saturate  UpperLimit=max(FLoadTor)  LowerLimit=0
  Scope{1..2,22..23,28} (5 alike) : Scope
  Scope26 : Scope  NumInputPorts=2
  Scope29 : Scope  NumInputPorts=2
  Subtract7 : Sum  Inputs=+++
  To Workspace2 : ToWorkspace  VariableName=W_engine_inp1  SaveFormat=Timeseries  SampleTime=-1
  FC (g) : Outport
  T_e_out (Nm) : Outport  Port=2
  W_e_out (rpm) : Outport  Port=3
  P_e (W) : Outport  Port=4
  wires:
  Motoring Torque Table1/1 -> Scope26/2, Subtract7/2  "T_e_motoring (Nm)"
  Integrator1/1 -> FC (g)/1, Scope28/1  "FC_tot"
  Derivative4/1 -> Gain23/1, Scope29/2  "w_e_dot (rad/s^2)"
  W_e_inp (rpm)/1 -> Gain24/1, W_e_out (rpm)/1, To Workspace2/1, Product8/2, FC Map1/2, 1-D Lookup Table1/2, Motoring Torque Table1/1, Scope23/1
  Product8/1 -> Gain21/1
  Tpos (0-1)/1 -> Scope22/1, 1-D Lookup Table1/1, FC Map1/1
  1-D Lookup Table1/1 -> Saturation6/1, Scope26/1  "T_e (Nm)"
  Gain24/1 -> Derivative4/1  "W_e (rad/s)"
  Gain23/1 -> Subtract7/3, Scope29/1  "T_e_inertia (Nm)"
  Gain21/1 -> P_e (W)/1  "P_e (W)"
  Gain22/1 -> Integrator1/1
  Subtract7/1 -> Scope1/1, T_e_out (Nm)/1, Product8/1  "T_e_out (Nm)"
  FC Map1/1 -> Gain22/1
  Saturation6/1 -> Subtract7/1
  ? -> Scope2/1

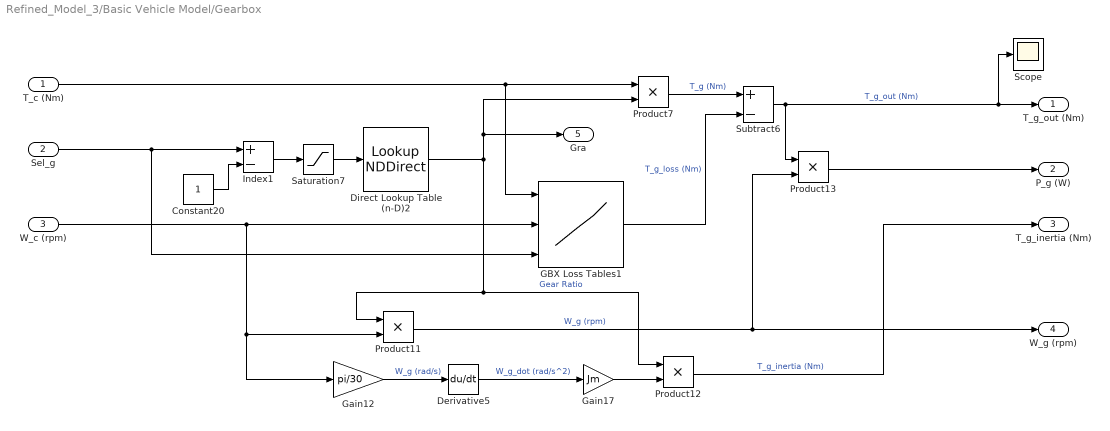
== system Refined_Model_3/Basic Vehicle Model/Gearbox ==
  T_c (Nm) : Inport
  Sel_g : Inport  Port=2
  W_c (rpm) : Inport  Port=3
  Constant20 : Constant
  Derivative5 : Derivative
  Direct Lookup Table (n-D)2 : LookupNDDirect  NumberOfTableDimensions=1  Table=GRa
  GBX Loss Tables1 : Lookup_n-D  NumberOfTableDimensions=3  BreakpointsForDimension1=GInpTor  BreakpointsForDimension2=GInprpm  BreakpointsForDimension3=GearNo  Table=GTorLoss  InterpMethod=Linear Lagrange  InternalRulePriority=Speed  RndMeth=Simplest  InputSameDT=on
      settings: InputPortMap=u0,u1,u2
  Gain12 : Gain  Gain=pi/30
  Gain17 : Gain  Gain=Jm
  Index1 : Sum  Inputs=+-
  Product{7,11..13} (4 alike) : Product
  Saturation7 : Saturate  UpperLimit=inf  LowerLimit=0
  Scope : Scope
  Subtract6 : Sum  Inputs=+-
  T_g_out (Nm) : Outport
  P_g (W) : Outport  Port=2
  T_g_inertia (Nm) : Outport  Port=3
  W_g (rpm) : Outport  Port=4
  Gra : Outport  Port=5
  wires:
  Product12/1 -> T_g_inertia (Nm)/1  "T_g_inertia (Nm)"
  Sel_g/1 -> GBX Loss Tables1/3, Index1/1
  Gain17/1 -> Product12/2
  T_c (Nm)/1 -> GBX Loss Tables1/1, Product7/1
  Product7/1 -> Subtract6/1  "T_g (Nm)"
  Product11/1 -> W_g (rpm)/1, Product13/2  "W_g (rpm)"
  Subtract6/1 -> Scope/1, T_g_out (Nm)/1, Product13/1  "T_g_out (Nm)"
  Derivative5/1 -> Gain17/1  "W_g_dot (rad/s^2)"
  Direct Lookup Table (n-D)2/1 -> Gra/1, Product7/2, Product11/1, Product12/1  "Gear Ratio"
  Saturation7/1 -> Direct Lookup Table (n-D)2/1
  Gain12/1 -> Derivative5/1  "W_g (rad/s)"
  Constant20/1 -> Index1/2
  GBX Loss Tables1/1 -> Subtract6/2  "T_g_loss (Nm)"
  Index1/1 -> Saturation7/1
  Product13/1 -> P_g (W)/1
  W_c (rpm)/1 -> GBX Loss Tables1/2, Gain12/1, Product11/2

== system Refined_Model_3/Basic Vehicle Model/If Action Subsystem3 ==
  In1 : Inport
  Action Port : ActionPort  ActionPortLabel=if(u1 < 3)
  Out1 : Outport
  wires:
  In1/1 -> Out1/1

== system Refined_Model_3/Basic Vehicle Model/If Action Subsystem4 ==
  In1 : Inport
  Action Port : ActionPort  ActionPortLabel=else
  Out1 : Outport
  wires:
  In1/1 -> Out1/1

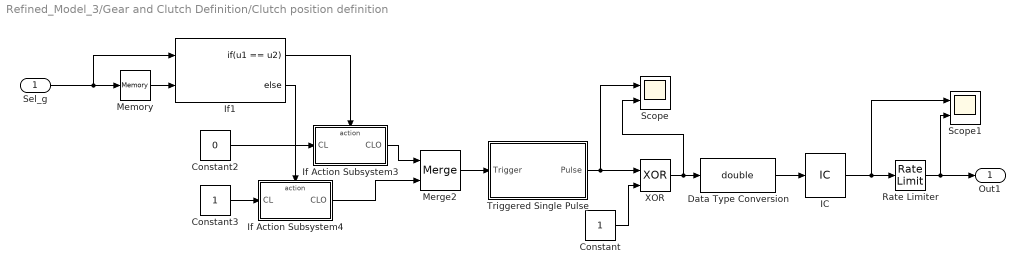
== system Refined_Model_3/Gear and Clutch Definition/Clutch position definition ==
  Sel_g : Inport
  Constant : Constant
  Constant2 : Constant  Value=0
  Constant3 : Constant
  Data Type Conversion : DataTypeConversion  OutDataTypeStr=double
  IC : InitialCondition  Value=0
  If Action Subsystem3 : Subsystem  TreatAsAtomicUnit=on
  If Action Subsystem4 : Subsystem  TreatAsAtomicUnit=on
  If1 : If  NumInputs=2  IfExpression=u1 == u2
  Memory : Memory
  Merge2 : Merge
  Rate Limiter : RateLimiter  RisingSlewLimit=0.5  FallingSlewLimit=-0.5  SampleTimeMode=inherited
  Scope : Scope  NumInputPorts=2
  Scope1 : Scope  NumInputPorts=2
  Triggered Single Pulse : Subsystem  TreatAsAtomicUnit=on  mask(single pulse generation){p_wid=1}
      mask prompts: p_wid "pulse width (number of samples)"
      mask help: This block generate a single pulse whenever a trigger happen. The pulse width must specified as a number of samples. for example if your sampling time is 0.1s and you want 3s pulse , then you should enter 30 as a pulse width.
      mask Display:
      | plot([0],[0])
      | plot([11],[0])
      | plot([5],[0.5])
      | plot([4 5 5 6 6 7],[0 0 0.25 0.25 0 0])
      | plot([5],[-0.3])
      | 
      | port_label('output', 1, 'Pulse')
      | port_label('input', 1, 'Trigger')
  XOR : Logic  Operator=XOR  IconShape=distinctive  AllPortsSameDT=off  OutDataTypeStr=boolean
  Out1 : Outport
  wires:
  If1/1 -> If Action Subsystem3/Action
  If Action Subsystem3/1(CLO) -> Merge2/1
  Memory/1 -> If1/2
  Constant2/1 -> If Action Subsystem3/1(CL)
  Constant3/1 -> If Action Subsystem4/1(CL)
  Sel_g/1 -> Memory/1, If1/1
  If1/2 -> If Action Subsystem4/Action
  If Action Subsystem4/1(CLO) -> Merge2/2
  Merge2/1 -> Triggered Single Pulse/1(Trigger)
  Triggered Single Pulse/1(Pulse) -> Scope/1, XOR/1
  Constant/1 -> XOR/2
  XOR/1 -> Scope/2, Data Type Conversion/1
  Data Type Conversion/1 -> IC/1
  Rate Limiter/1 -> Out1/1, Scope1/2
  IC/1 -> Scope1/1, Rate Limiter/1

== system Refined_Model_3/Gear and Clutch Definition/If Action Subsystem ==
  In1 : Inport
  Action Port : ActionPort  ActionPortLabel=if(u1 > 2.8)
  Out1 : Outport
  wires:
  In1/1 -> Out1/1

== system Refined_Model_3/Gear and Clutch Definition/If Action Subsystem1 ==
  In1 : Inport
  Action Port : ActionPort  ActionPortLabel=elseif(u1 > 5.5)
  Out1 : Outport
  wires:
  In1/1 -> Out1/1

== system Refined_Model_3/Gear and Clutch Definition/If Action Subsystem2 ==
  In1 : Inport
  Action Port : ActionPort  ActionPortLabel=else
  Out1 : Outport
  wires:
  In1/1 -> Out1/1

== system Refined_Model_3/Gear and Clutch Definition/If Action Subsystem3 ==
  Selected Gear /dt : Inport
  Action Port : ActionPort  ActionPortLabel=if(u1 >= u2 & u3 < u4)
  Add : Sum
  Constant : Constant
  Increased gear : Outport
  wires:
  Selected Gear /dt/1 -> Add/1
  Add/1 -> Increased gear/1
  Constant/1 -> Add/2

== system Refined_Model_3/Gear and Clutch Definition/If Action Subsystem4 ==
  Selected Gear /dt : Inport
  Action Port : ActionPort  ActionPortLabel=elseif(u3 >= u4 & u1 < u2)
  Constant : Constant
  Subtract : Sum  Inputs=+-
  Decreased gear : Outport
  wires:
  Constant/1 -> Subtract/2
  Subtract/1 -> Decreased gear/1
  Selected Gear /dt/1 -> Subtract/1

== system Refined_Model_3/Gear and Clutch Definition/If Action Subsystem5 ==
  Selected Gear Ratio /dt : Inport
  Action Port : ActionPort  ActionPortLabel=else
  Out1 : Outport
  wires:
  Selected Gear Ratio /dt/1 -> Out1/1

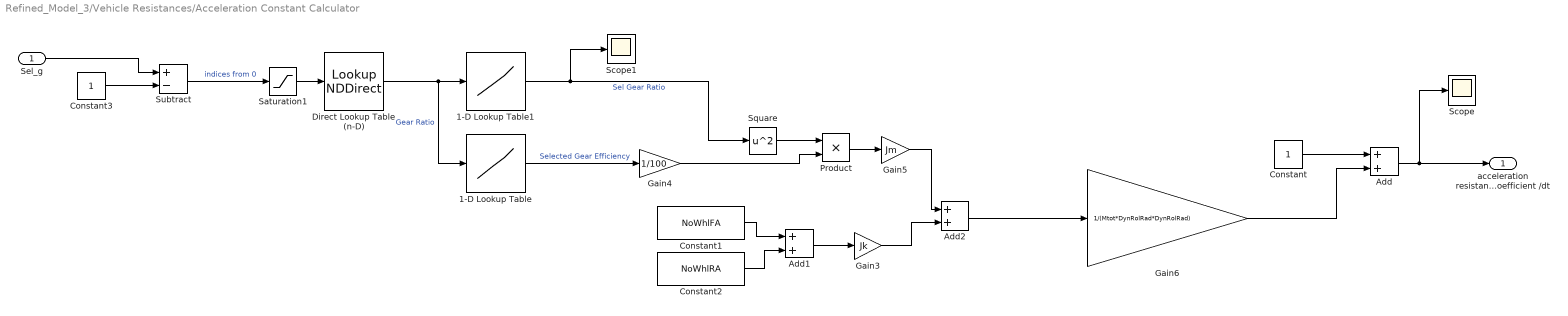
== system Refined_Model_3/Vehicle Resistances/Acceleration Constant Calculator ==
  Sel_g : Inport
  1-D Lookup Table : Lookup_n-D  NumberOfTableDimensions=1  BreakpointsForDimension1=GNo  Table=etaGRa  InternalRulePriority=Speed  RndMeth=Simplest  InputSameDT=on
  1-D Lookup Table1 : Lookup_n-D  NumberOfTableDimensions=1  BreakpointsForDimension1=GNo  Table=GRa  InternalRulePriority=Speed  RndMeth=Simplest  InputSameDT=on
  Add : Sum
  Add1 : Sum
  Add2 : Sum
  Constant : Constant
  Constant1 : Constant  Value=NoWhlFA
  Constant2 : Constant  Value=NoWhlRA
  Constant3 : Constant
  Direct Lookup Table (n-D) : LookupNDDirect  NumberOfTableDimensions=1  Table=GRa
  Gain3 : Gain  Gain=Jk
  Gain4 : Gain  Gain=1/100
  Gain5 : Gain  Gain=Jm
  Gain6 : Gain  Gain=1/(Mtot*DynRolRad*DynRolRad)
  Product : Product
  Saturation1 : Saturate  UpperLimit=inf  LowerLimit=0
  Scope : Scope
  Scope1 : Scope
  Square : Math  Operator=square  SaturateOnIntegerOverflow=on
  Subtract : Sum  Inputs=+-
  acceleration resistance coefficient /dt : Outport
  wires:
  1-D Lookup Table/1 -> Gain4/1  "Selected Gear Efficiency"
  Add1/1 -> Gain3/1
  Product/1 -> Gain5/1
  Gain6/1 -> Add/2
  Square/1 -> Product/1
  Constant2/1 -> Add1/2
  Constant/1 -> Add/1
  Gain3/1 -> Add2/2
  Add2/1 -> Gain6/1
  Constant1/1 -> Add1/1
  Gain4/1 -> Product/2
  Gain5/1 -> Add2/1
  1-D Lookup Table1/1 -> Scope1/1, Square/1  "Sel Gear Ratio"
  Add/1 -> Scope/1, acceleration resistance coefficient /dt/1
  Saturation1/1 -> Direct Lookup Table (n-D)/1
  Subtract/1 -> Saturation1/1  "indices from 0"
  Constant3/1 -> Subtract/2
  Direct Lookup Table (n-D)/1 -> 1-D Lookup Table/1, 1-D Lookup Table1/1  "Gear Ratio"
  Sel_g/1 -> Subtract/1

== system Refined_Model_3/Vehicle Resistances/If Action Subsystem ==
  In1 : Inport
  Action Port : ActionPort  ActionPortLabel=if(u1 > 0)
  Out1 : Outport
  wires:
  In1/1 -> Out1/1

== system Refined_Model_3/Vehicle Resistances/If Action Subsystem1 ==
  In1 : Inport
  Action Port : ActionPort  ActionPortLabel=else
  Out1 : Outport
  wires:
  In1/1 -> Out1/1

== system Refined_Model_3/Acc//Dec Control/Look Ahead Braking Model/If Action Subsystem ==
  In : Inport
  Action Port : ActionPort  ActionPortLabel=if(u1 > 0)
  Out1 : Outport
  wires:
  In/1 -> Out1/1  "deceleration in m/s^2"

== system Refined_Model_3/Acc//Dec Control/Look Ahead Braking Model/If Action Subsystem1 ==
  In1 : Inport
  Action Port : ActionPort  ActionPortLabel=else
  Out1 : Outport
  wires:
  In1/1 -> Out1/1

== system Refined_Model_3/Acc//Dec Control/Look Ahead Braking Model/If Action Subsystem2 ==
  In1 : Inport
  Action Port : ActionPort  ActionPortLabel=if(u1 <= u2 & u3 < u4)
  Out1 : Outport
  wires:
  In1/1 -> Out1/1

== system Refined_Model_3/Acc//Dec Control/Look Ahead Braking Model/If Action Subsystem3 ==
  In1 : Inport
  Action Port : ActionPort  ActionPortLabel=else
  Out1 : Outport
  wires:
  In1/1 -> Out1/1

== system Refined_Model_3/Basic Vehicle Model/Chassis/Trip complete2 ==
  Disp (m) : Inport
  Constant1 : Constant  Value=NoSteps
  Constant2 : Constant
  If : If  NumInputs=2  IfExpression=u1 > u2  ShowElse=off
  If Action Subsystem : Subsystem  TreatAsAtomicUnit=on
  Stop Simulation : Stop
  wires:
  Constant1/1 -> If/2
  Constant2/1 -> If Action Subsystem/1(In1)
  If/1 -> If Action Subsystem/Action
  If Action Subsystem/1(Out1) -> Stop Simulation/1
  Disp (m)/1 -> If/1

== system Refined_Model_3/Gear and Clutch Definition/Clutch position definition/If Action Subsystem3 ==
  CL : Inport
  Action Port : ActionPort  ActionPortLabel=if(u1 == u2)
  CLO : Outport
  wires:
  CL/1 -> CLO/1

== system Refined_Model_3/Gear and Clutch Definition/Clutch position definition/If Action Subsystem4 ==
  CL : Inport
  Action Port : ActionPort  ActionPortLabel=else
  CLO : Outport
  wires:
  CL/1 -> CLO/1

== system Refined_Model_3/Gear and Clutch Definition/Clutch position definition/Triggered Single Pulse ==
  Trigger : Inport
  +ve edge detect : Subsystem
  Add : Sum
  Add1 : Sum
  Compare To Constant : simulink/Logic and Bit Operations/Compare To Constant  relop=>  const=p_wid-1  OutDataTypeStr=boolean
  Constant2 : Constant
  Logical Operator : Logic  Operator=NOT  AllPortsSameDT=off  OutDataTypeStr=boolean
  Product : Product  RndMeth=Zero
  Product1 : Product  RndMeth=Zero
  Product3 : Product  RndMeth=Zero
  Saturation : Saturate  UpperLimit=1  LowerLimit=0
  Unit Delay : UnitDelay  SampleTime=-1  HasFrameUpgradeWarning=on
  Unit Delay1 : UnitDelay  SampleTime=-1  HasFrameUpgradeWarning=on
  Pulse : Outport
  wires:
  Compare To Constant/1 -> Logical Operator/1
  Constant2/1 -> Product/1
  Product/1 -> Add/1
  Unit Delay/1 -> Add/2, Compare To Constant/1
  Trigger/1 -> +ve edge detect/1(signal)
  +ve edge detect/1(out) -> Add1/2
  Add/1 -> Product1/2
  Product1/1 -> Unit Delay/1
  Add1/1 -> Unit Delay1/1
  Unit Delay1/1 -> Saturation/1
  Saturation/1 -> Product3/1
  Product3/1 -> Add1/1, Product/2, Product1/1, Pulse/1
  Logical Operator/1 -> Product3/2

== system Refined_Model_3/Basic Vehicle Model/Chassis/Trip complete2/If Action Subsystem ==
  In1 : Inport
  Action Port : ActionPort  ActionPortLabel=if(u1 > u2)
  Out1 : Outport
  wires:
  In1/1 -> Out1/1

== system Refined_Model_3/Gear and Clutch Definition/Clutch position definition/Triggered Single Pulse/+ve edge detect ==
  note: Edge
  signal : Inport
  Delay Input1 : UnitDelay  Description=Store in Global RAM  DisableCoverage=on  SampleTime=-1  HasFrameUpgradeWarning=on
  FixPt Relational Operator : RelationalOperator  Operator=>  OutDataTypeStr=fixdt(0, 8)  ZeroCross=off  RndMeth=Nearest
  Positive : simulink/Logic and Bit Operations/Compare To Zero  relop=>  OutDataTypeStr=uint8  ZeroCross=off
  out : Outport
  wires:
  Delay Input1/1 -> FixPt Relational Operator/2  "U(k-1)"
  Positive/1 -> Delay Input1/1, FixPt Relational Operator/1  "U(k)"
  FixPt Relational Operator/1 -> out/1
  signal/1 -> Positive/1
